simulink model "reg_neuronowy"  (R2017b)
settings: Solver=VariableStepAuto  StartTime=0.0  StopTime=10.0  RelTol=1e-3
libraries: neural x6
settings Model: Creator=kamil  LastModifiedBy=kamil

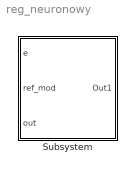
== system reg_neuronowy ==
  Subsystem : Subsystem

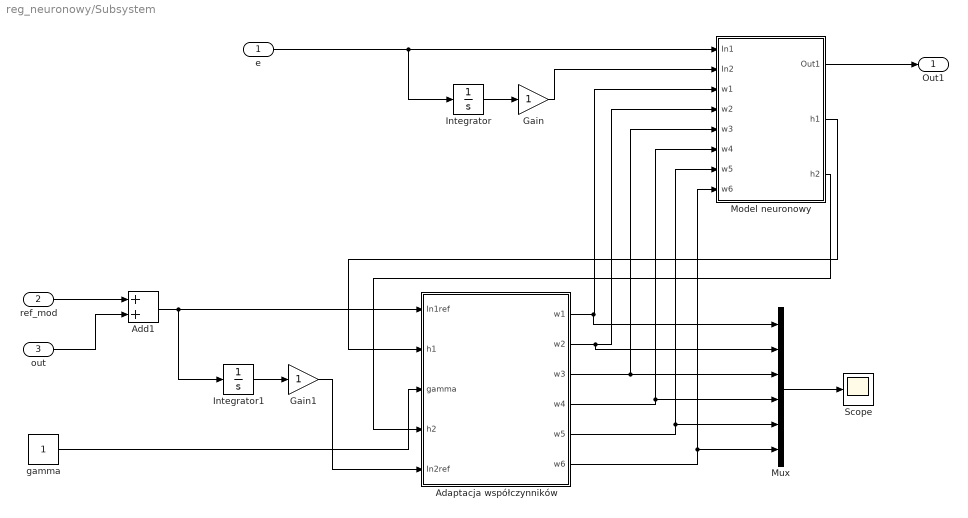
== system reg_neuronowy/Subsystem ==
  e : Inport
  ref_mod : Inport  Port=2
  out : Inport  Port=3
  Adaptacja współczynników : Subsystem
  Add1 : Sum
  Gain : Gain
  Gain1 : Gain
  Integrator : Integrator
  Integrator1 : Integrator
  Model neuronowy : Subsystem
  Mux : Mux  Inputs=6
  Scope : Scope
  gamma : Constant
  Out1 : Outport
  wires:
  Adaptacja współczynników/6(w6) -> Mux/6, Model neuronowy/8(w6)
  gamma/1 -> Adaptacja współczynników/3(gamma)
  Mux/1 -> Scope/1
  Model neuronowy/2(h1) -> Adaptacja współczynników/2(h1)
  Adaptacja współczynników/5(w5) -> Mux/5, Model neuronowy/7(w5)
  Integrator1/1 -> Gain1/1
  Add1/1 -> Integrator1/1, Adaptacja współczynników/1(In1ref)
  Gain1/1 -> Adaptacja współczynników/5(In2ref)
  Gain/1 -> Model neuronowy/2(In2)
  Adaptacja współczynników/3(w3) -> Mux/3, Model neuronowy/5(w3)
  ref_mod/1 -> Add1/1
  Adaptacja współczynników/4(w4) -> Mux/4, Model neuronowy/6(w4)
  Adaptacja współczynników/1(w1) -> Mux/1, Model neuronowy/3(w1)
  Adaptacja współczynników/2(w2) -> Mux/2, Model neuronowy/4(w2)
  Model neuronowy/3(h2) -> Adaptacja współczynników/4(h2)
  out/1 -> Add1/2
  e/1 -> Integrator/1, Model neuronowy/1(In1)
  Integrator/1 -> Gain/1
  Model neuronowy/1(Out1) -> Out1/1

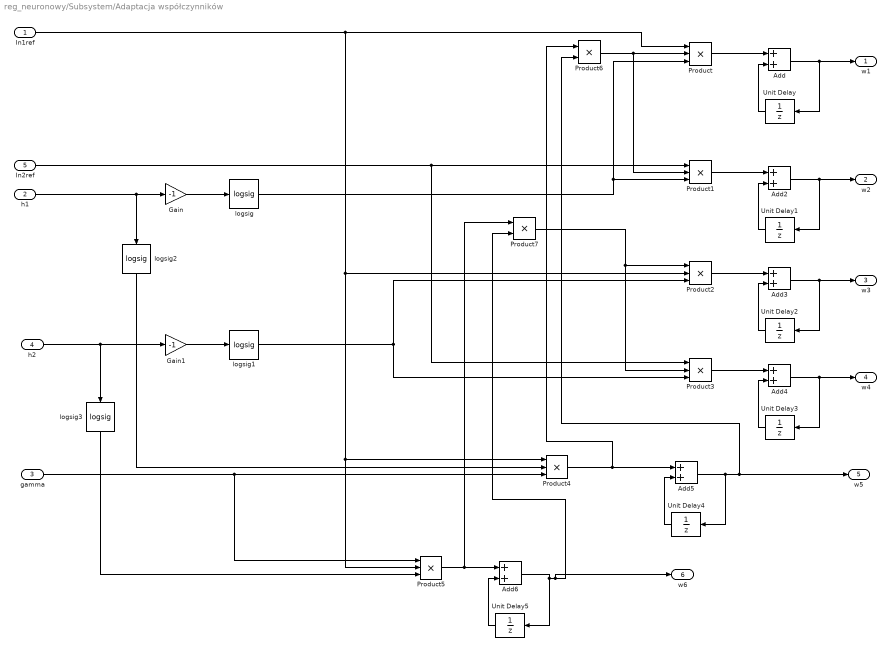
== system reg_neuronowy/Subsystem/Adaptacja współczynników ==
  In1ref : Inport
  h1 : Inport  Port=2
  gamma : Inport  Port=3
  h2 : Inport  Port=4
  In2ref : Inport  Port=5
  Add{,2..6} (6 alike) : Sum
  Gain : Gain  Gain=-1
  Gain1 : Gain  Gain=-1
  Product{,1..5} (6 alike) : Product  Inputs=3
  Product6 : Product
  Product7 : Product
  Unit Delay{,1..5} (6 alike) : UnitDelay  SampleTime=-1
  logsig{,1..3} (4 alike) : neural/Transfer Functions/logsig
      settings: SourceProductName=Neural Network Toolbox  SourceProductBaseCode=NN
  w1 : Outport
  w2 : Outport  Port=2
  w3 : Outport  Port=3
  w4 : Outport  Port=4
  w5 : Outport  Port=5
  w6 : Outport  Port=6
  wires:
  Product7/1 -> Product3/2, Product2/1
  Gain/1 -> logsig/1
  h2/1 -> logsig3/1, Gain1/1
  logsig1/1 -> Product3/3, Product2/3
  In1ref/1 -> Product/1, Product2/2, Product4/1, Product5/2
  Unit Delay1/1 -> Add2/2
  Unit Delay3/1 -> Add4/2
  Product2/1 -> Add3/1
  Unit Delay/1 -> Add/2
  Add/1 -> w1/1, Unit Delay/1
  Product/1 -> Add/1
  Add4/1 -> w4/1, Unit Delay3/1
  Add5/1 -> w5/1, Product6/2, Unit Delay4/1
  Product5/1 -> Product7/1, Add6/1
  Unit Delay5/1 -> Add6/2
  Add3/1 -> w3/1, Unit Delay2/1
  Product6/1 -> Product1/2, Product/2
  Unit Delay2/1 -> Add3/2
  Add2/1 -> w2/1, Unit Delay1/1
  gamma/1 -> Product5/1, Product4/3
  Add6/1 -> w6/1, Product7/2, Unit Delay5/1
  Unit Delay4/1 -> Add5/2
  Product1/1 -> Add2/1
  Product4/1 -> Product6/1, Add5/1
  Product3/1 -> Add4/1
  Gain1/1 -> logsig1/1
  logsig2/1 -> Product4/2
  logsig3/1 -> Product5/3
  In2ref/1 -> Product3/1, Product1/1
  logsig/1 -> Product1/3, Product/3
  h1/1 -> logsig2/1, Gain/1

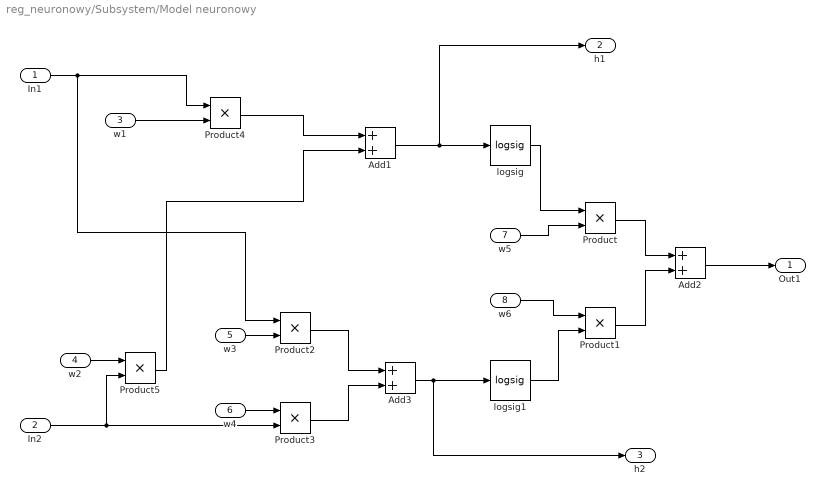
== system reg_neuronowy/Subsystem/Model neuronowy ==
  In1 : Inport
  In2 : Inport  Port=2
  w1 : Inport  Port=3
  w2 : Inport  Port=4
  w3 : Inport  Port=5
  w4 : Inport  Port=6
  w5 : Inport  Port=7
  w6 : Inport  Port=8
  Add1 : Sum
  Add2 : Sum
  Add3 : Sum
  Product{,1..5} (6 alike) : Product
  logsig : neural/Transfer Functions/logsig
      settings: SourceProductName=Neural Network Toolbox  SourceProductBaseCode=NN
  logsig1 : neural/Transfer Functions/logsig
      settings: SourceProductName=Neural Network Toolbox  SourceProductBaseCode=NN
  Out1 : Outport
  h1 : Outport  Port=2
  h2 : Outport  Port=3
  wires:
  Add1/1 -> h1/1, logsig/1
  Product1/1 -> Add2/2
  w4/1 -> Product3/1
  Add3/1 -> h2/1, logsig1/1
  w6/1 -> Product1/1
  w3/1 -> Product2/2
  In1/1 -> Product2/1, Product4/1
  w1/1 -> Product4/2
  w2/1 -> Product5/1
  In2/1 -> Product5/2, Product3/2
  Product4/1 -> Add1/1
  Add2/1 -> Out1/1
  Product3/1 -> Add3/2
  Product2/1 -> Add3/1
  logsig/1 -> Product/1
  Product5/1 -> Add1/2
  logsig1/1 -> Product1/2
  w5/1 -> Product/2
  Product/1 -> Add2/1
